simulink model "ADC_personal_2"  (R2024a)
settings: Solver=VariableStepAuto  StartTime=0.0  StopTime=10e-5  RelTol=1e-3
PreLoadFcn:
  | jitter = 145e-15
StopFcn:
  | dy = yout - mean(yout);
  | rmsjitter = std(dy);
  | histogram(dy,50);
  | title(['\bfjitter didtribution: RMS jitter = ',num2str(rmsjitter),'s']);
  | xlabel('Time (s) -->');
  | ylabel('Occurances (count) -->');
libraries: dspfdesign x2
settings Model: Creator=GILBERT KELECHI  LastModifiedBy=GILBERT KELECHI

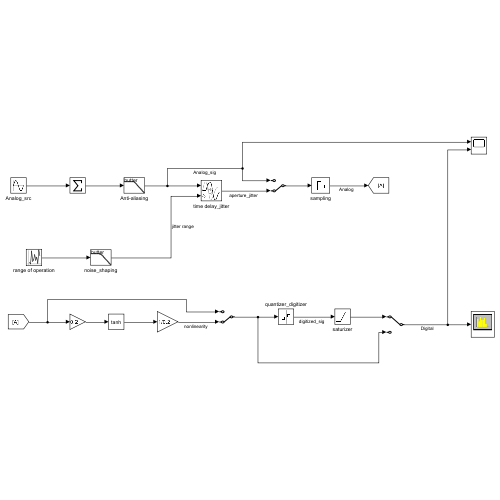
[thumbnail: Simulink's stored preview of the top-level diagram]
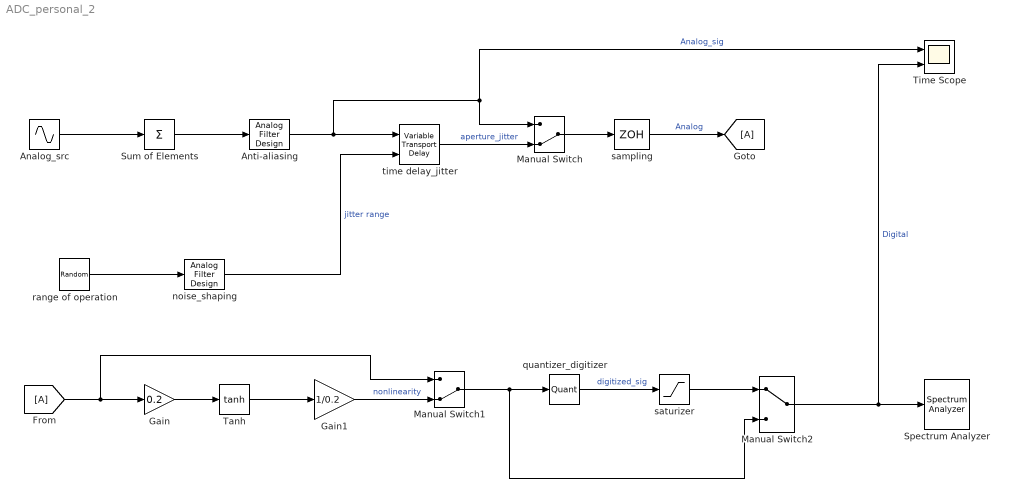
== system ADC_personal_2 ==
  Analog_src : Sin  Amplitude=0.25  Frequency=2*pi*[20 22]*1e6  SampleTime=0
  Anti-aliasing : dspfdesign/Analog Filter Design  method=Butterworth  filttype=Lowpass  N=8  Wlo=2*pi*50e6  Whi=80  Rp=2  Rs=40
  From : From
  Gain : Gain  Gain=0.2
  Gain1 : Gain  Gain=1/0.2
  Goto : Goto
  Manual Switch : ManualSwitch  CurrentSetting=0
  Manual Switch1 : ManualSwitch  CurrentSetting=0
  Manual Switch2 : ManualSwitch
  Spectrum Analyzer : SpectrumAnalyzer  WindowPosition=[997.000000,50.000000,847.000000,526.000000,]  ScopeFrameLocation=window  SampleRateSource=Property  SampleRate=44.1e3  PlotAsTwoSidedSpectrum=off  FrequencySpan=Start and stop frequencies  StartFrequency=20  StopFrequency=20e3  SelectedToolstripTab=spectrumAnalyzerToolstrip.spectrumTab
  Sum of Elements : Sum  Inputs=+
  Tanh : Trigonometry  Operator=tanh
  Time Scope : Scope  NumInputPorts=2
  noise_shaping : dspfdesign/Analog Filter Design  method=Butterworth  filttype=Lowpass  N=3  Wlo=2*pi*20e+06  Whi=80  Rp=2  Rs=40
  quantizer_digitizer : Quantizer  QuantizationInterval=2^-12
  range of operation : UniformRandomNumber  Minimum=0  Maximum=5e-9  Seed=1234  SampleTime=0
  sampling : ZeroOrderHold  SampleTime=1/100e6
  saturizer : Saturate
  time delay_jitter : VariableTransportDelay  MaximumDelay=30e-9  ZeroDelay=on  TransDelayFeedthrough=on
  wires:
  Analog_src/1 -> Sum of Elements/1
  Sum of Elements/1 -> Anti-aliasing/1
  Anti-aliasing/1 -> Time Scope/1, Manual Switch/1, time delay_jitter/1  "Analog_sig"
  range of operation/1 -> noise_shaping/1
  noise_shaping/1 -> time delay_jitter/2  "jitter range"
  time delay_jitter/1 -> Manual Switch/2  "aperture_jitter"
  Manual Switch/1 -> sampling/1
  sampling/1 -> Goto/1  "Analog"
  From/1 -> Manual Switch1/1, Gain/1
  Gain/1 -> Tanh/1
  Tanh/1 -> Gain1/1
  Gain1/1 -> Manual Switch1/2  "nonlinearity"
  Manual Switch1/1 -> Manual Switch2/2, quantizer_digitizer/1
  quantizer_digitizer/1 -> saturizer/1  "digitized_sig"
  saturizer/1 -> Manual Switch2/1
  Manual Switch2/1 -> Time Scope/2, Spectrum Analyzer/1  "Digital"
